simulink library "sunVector_lib"  (R2018b)
settings: Solver=VariableStepAuto  StartTime=0.0  StopTime=10.0  RelTol=1e-3
settings Model: Creator=devantormey  LastModifiedBy=taylorreynolds

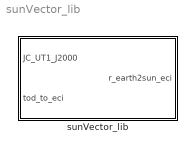
== system sunVector_lib ==
  sunVector_lib : Subsystem

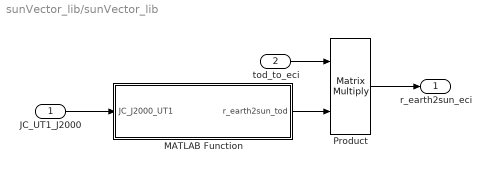
== system sunVector_lib/sunVector_lib ==
  JC_UT1_J2000 : Inport
  tod_to_eci : Inport  Port=2
  MATLAB Function : MATLAB Function  TreatAsAtomicUnit=on
  Product : Product  Multiplication=Matrix(*)
  r_earth2sun_eci : Outport
  wires:
  MATLAB Function/1(r_earth2sun_tod) -> Product/2
  JC_UT1_J2000/1 -> MATLAB Function/1(JC_J2000_UT1)
  tod_to_eci/1 -> Product/1
  Product/1 -> r_earth2sun_eci/1

== matlab function sunVector_lib/MATLAB Function ==
  data: JC_J2000_UT1 input; r_earth2sun_tod output
function r_earth2sun_tod = sun(JC_J2000_UT1)
%SUN 
%
% This function computes the vector position of the sun relative to Earth
% in the TOD (true-of-date) frame.
%
% Inputs:
%   - JC_J2000_UT1 [scalar, double] : current datetime in Julian Centuries
%   referenced to the J2000 epoch, in the UT1 frame
% 
% Ouputs:
%   - r_earth2sun [3x1, double] : current vector from the center of the
%   Earth to the center of the sun in the TOD coordinate frame
%
% Reference: Vallado 4e pp. 277-280 (see Algorithm 29)
%   - see also the errata for this page range re. the change to TOD
%
% T. P. Reynolds (08.26.20)
%#codegen
deg2rad = pi/180.0;

% first compute mean longitude
phi_s = 280.460 + 36000.77 * JC_J2000_UT1;        % [deg]
phi_s = mod( deg2rad*phi_s, 2*pi);                % [rad]
% Now compute mean anomoly using JC_J2000_UT1 approx JC_J2000_TDB
M_s = 357.5277233 + 35999.05034 * JC_J2000_UT1;   % [deg]
M_s = mod( deg2rad*M_s, 2*pi);                    % [rad]

% now compute longitude of the ecliptic using
phi_e = phi_s + (deg2rad*1.914666471) * sin(M_s) ...
              + (deg2rad*0.019994643) * sin(2*M_s);  % [rad]

% Obliquity of ecliptic
eps = deg2rad * (23.439291 - 0.0130042 * JC_J2000_UT1);             % [rad]

% compute magnitude of earth-to-sun vector
r = 1.000140612 - 0.016708617 * cos(M_s) - 0.000139589 * cos(2*M_s); % [Au]

% compute earth-to-sun vector 
r_earth2sun_tod = r.* [ cos(phi_e);
                        cos(eps)*sin(phi_e); 
                        sin(eps)*sin(phi_e) ];
end
